simulink model "problem5"  (R2020a)
settings: Solver=VariableStepAuto  StartTime=0.0  StopTime=10.0  RelTol=1e-3
model workspace (MAT data in the model file):
  C = Simulink.Parameter
  C.Value = 1e-06
  C.DataType = 'auto'
  C.Dimensions = [1 1]
  R = Simulink.Parameter
  R.Value = 10
  R.DataType = 'auto'
  R.Dimensions = [1 1]
values from neighbouring files (symbols this model uses):
  C = 10^(-6)    (= 1e-06)    [Problem5.m]    (also in problem5.mat)
  R = 10    [Problem5.m]    (also in problem5.mat)
settings Model: Creator=HP  LastModifiedBy=HP

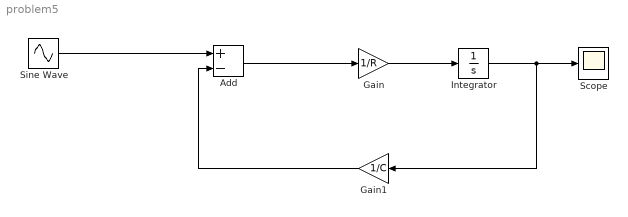
== system problem5 ==
  Add : Sum  Inputs=+-
  Gain : Gain  Gain=1/R
  Gain1 : Gain  Gain=1/C
  Integrator : Integrator
  Scope : Scope
  Sine Wave : Sin  Amplitude=2  Frequency=2*pi  SampleTime=0
  wires:
  Sine Wave/1 -> Add/1
  Integrator/1 -> Gain1/1, Scope/1
  Add/1 -> Gain/1
  Gain1/1 -> Add/2
  Gain/1 -> Integrator/1
